simulink model "simulation"  (R2024a)
settings: Solver=VariableStepAuto  StartTime=0.0  StopTime=50  RelTol=1e-3
values from neighbouring files (symbols this model uses):
  A = expm(A*T)    [benchmark_project.m]
  B = (eye(4)*T + A*T^2/2 + A^2*T^3/6 + A^3*T^4/24)*B    [benchmark_project.m]
  C = [0 0 1 0]    [benchmark_project.m]
  G = kalman_gains{N}    [benchmark_project.m]
  K = K{1}    [benchmark_project.m]
  q0 = [0;0;0;0]    [benchmark_project.m]
  T = .01    (= 0.01)    [benchmark_project.m]
  x0 = [0;0;0;0]    [benchmark_project.m]
settings Model: Creator=Zargai  LastModifiedBy=Zargai

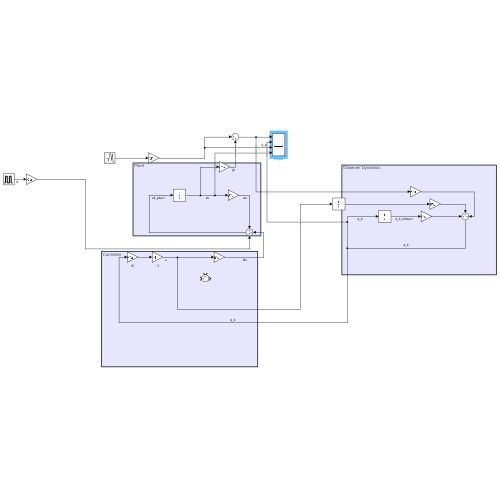
[thumbnail: Simulink's stored preview of the top-level diagram]
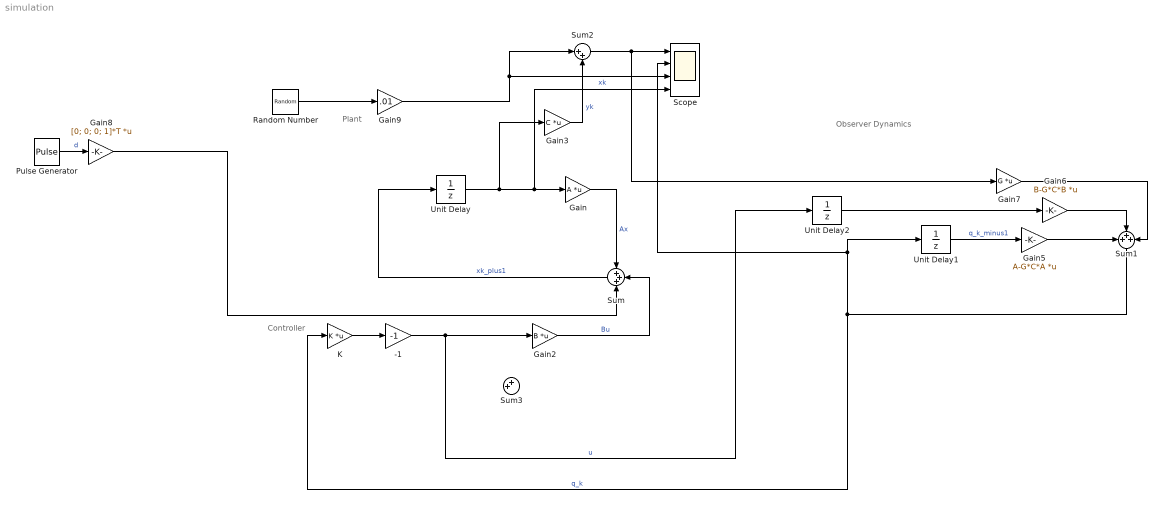
== system simulation ==
  note: Observer Dynamics
  note: Controller
  note: Plant
  -1 : Gain  Gain=-1
  Gain : Gain  Gain=A  Multiplication=Matrix(K*u)
  Gain2 : Gain  Gain=B  Multiplication=Matrix(K*u)
  Gain3 : Gain  Gain=C  Multiplication=Matrix(K*u)
  Gain5 : Gain  Gain=A-G*C*A  Multiplication=Matrix(K*u)
  Gain6 : Gain  Gain=B-G*C*B  Multiplication=Matrix(K*u)
  Gain7 : Gain  Gain=G  Multiplication=Matrix(K*u)
  Gain8 : Gain  Gain=[0; 0; 0; 1]*T  Multiplication=Matrix(K*u)
  Gain9 : Gain  Gain=.01
  K : Gain  Gain=K  Multiplication=Matrix(K*u)
  Pulse Generator : DiscretePulseGenerator  PulseType=Time based  Period=100
  Random Number : RandomNumber  Variance=20  SampleTime=T
  Scope : Scope  NumInputPorts=4
  Sum : Sum  Inputs=+++
  Sum1 : Sum  Inputs=+++
  Sum2 : Sum  Inputs=|++
  Sum3 : Sum  Inputs=++|
  Unit Delay : UnitDelay  InitialCondition=x0  SampleTime=T  HasFrameUpgradeWarning=on
  Unit Delay1 : UnitDelay  InitialCondition=q0  SampleTime=T  HasFrameUpgradeWarning=on
  Unit Delay2 : UnitDelay  SampleTime=T  HasFrameUpgradeWarning=on
  wires:
  Sum/1 -> Unit Delay/1  "xk_plus1"
  Unit Delay/1 -> Gain3/1, Scope/4, Gain/1  "xk"
  Gain/1 -> Sum/1  "Ax"
  Gain3/1 -> Sum2/2  "yk"
  Gain2/1 -> Sum/2  "Bu"
  K/1 -> -1/1
  Sum1/1 -> Scope/2, Unit Delay1/1, K/1  "q_k"
  Unit Delay1/1 -> Gain5/1  "q_k_minus1"
  Gain5/1 -> Sum1/1
  Gain6/1 -> Sum1/2
  Gain7/1 -> Sum1/3
  Unit Delay2/1 -> Gain6/1
  Random Number/1 -> Gain9/1
  Gain9/1 -> Sum2/1, Scope/3
  Sum2/1 -> Gain7/1, Scope/1
  Pulse Generator/1 -> Gain8/1  "d"
  -1/1 -> Unit Delay2/1, Gain2/1  "u"
  Gain8/1 -> Sum/3
